simulink model "sampleModel1535"  (R2023a)
settings: Solver=VariableStepAuto  StartTime=0.0  StopTime=10.0  RelTol=1e-3
libraries: simulink x3, hdlsllib x2
settings Model: Creator=user1  LastModifiedBy=user1

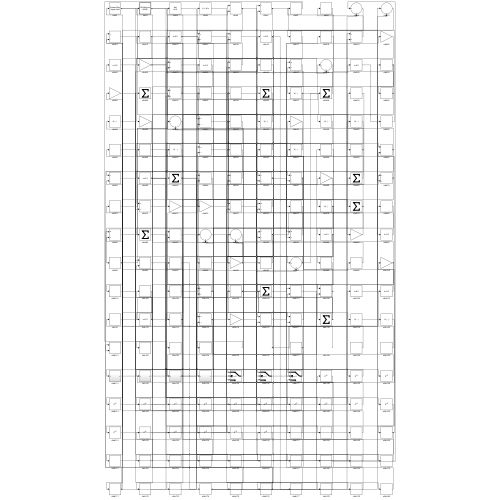
[thumbnail: Simulink's stored preview of the top-level diagram]
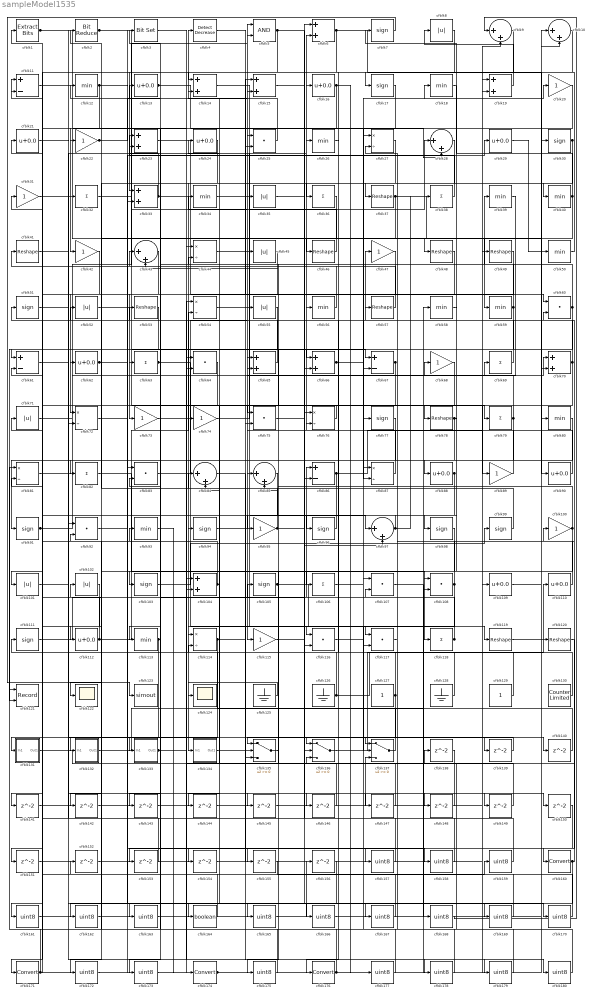
== system sampleModel1535 ==
  cfblk1 : simulink/Logic and Bit Operations/Extract Bits  bitsToExtract=Upper half  numBits=8  bitIdxRange=[0 7]  outScalingMode=Preserve fixed-point scaling
      settings: LibrarySourceBlock=|
      | hdlsllib/Logic and Bit
      | Operations/Extract Bits
  cfblk{9..10,28,43,84..85,97} (7 alike) : Sum  Inputs=|++
  cfblk{20,22,31,42,47,68,73..74,89,95,100,115} (12 alike) : Gain
  cfblk{8,35,45,52,55,71,101..102} (8 alike) : Abs  SaturateOnIntegerOverflow=off
  cfblk{7,17,30,51,77,91,94,96,98..99,103,105,111} (13 alike) : Signum
  cfblk{6,14..15,19,23,33,65..66,70,104} (10 alike) : Sum
  cfblk{32,36,38,63,69,79,82,106,118} (9 alike) : Sum  Inputs=+
  cfblk{25,60,64,75,83,92,107..108,116..117} (10 alike) : DotProduct  OutDataTypeStr=Inherit: Inherit via internal rule
  cfblk{13,16,21,24,29,62,88,90,109..110,112} (11 alike) : Bias  Bias=0.0  SaturateOnIntegerOverflow=off
  cfblk{11,61,67,86} (4 alike) : Sum  Inputs=+-
  cfblk{12,18,26,34,39..40,50,56,58..59,80,93,113} (13 alike) : MinMax
  cfblk{27,44,54,72,76,81,87,114} (8 alike) : Product  Inputs=*/  RndMeth=Zero  SaturateOnIntegerOverflow=on
  cfblk{37,41,46,48..49,53,57,78,119..120} (10 alike) : Reshape
  cfblk121 : Record  FileSettingsInternal="{\"entries\":[{\"content\":{\"excelSettings\":{\"content\":{},\"type\":\"Streamout.ExcelSettings\"}},\"type\":\"Streamout.FileSettingStorage\",\"uuid\":\"\"}],\"packageUris\":[\"http:\\/\\/schema.mathworks.com\\/mf0\\/streamout_blocks\\/R2020a\"],\"version\":\"1.0\"}"  Layout=[1 1]  SignalsInternal="{\"entries\":[{\"content\":{\"signals\":[{\"content\":{\"blockPath\":[],\"dimensions\":[1],\"domain\":\"\",\"lineColor\":\"#a2142f\",\"plots\":[1],\"port\":1,\"signalID\":1564,\"signalName\":\"XY Graph:1\"},\"type\":\"RecordBlkView.Signal\",\"uuid\":\"\"},{\"content\":{\"blockPath\":[],\"dimensions\":[1],\"domain\":\"\",\"lineColor\":\"#139fff\",\"plots\":[1],\"port\":2,\"signalID\":1567,\"signalName\":\"XY Graph:2\"},\"type\":\"RecordBlkView.Signal\",\"uuid\":\"\"}]},\"type\":\"RecordBlkView.InputSignals\",\"uuid\":\"\"}],\"packageUris\":[\"http:\\/\\/schema.mathworks.com\\/mf0\\/streamout_blocks\\/R2020a\"],\"version\":\"1.0\"}"  VisualizationBindings="{\"xyplotplugin\":{\"info\":[{\"series\":[{\"bindingParametersList\":[{\"parameter\":\"X-Axis\",\"signalID\":1564,\"signalName\":\"XY Graph:1\"},{\"parameter\":\"Y-Axis\",\"signalID\":1567,\"signalName\":\"XY Graph:2\"}],\"seriesID\":27336}],\"subplotID\":1}]}}"  CompatibilityTag=XY  st=-1
  cfblk122 : Scope
  cfblk123 : ToWorkspace  VariableName=simout  SaveFormat=Timeseries  SampleTime=-1
  cfblk124 : Scope
  cfblk125 : Ground
  cfblk126 : Ground
  cfblk127 : Constant  SampleTime=-1
  cfblk128 : Ground
  cfblk129 : Constant  SampleTime=-1
  cfblk130 : hdlsllib/Sources/Counter Limited  uplimit=7  tsamp=-1
  cfblk131 : Subsystem
      settings: LibrarySourceBlock=|
      | hdlsllib/Ports &
      | Subsystems/Subsystem
  cfblk132 : Subsystem
      settings: LibrarySourceBlock=|
      | hdlsllib/Ports &
      | Subsystems/Subsystem
  cfblk133 : Subsystem
      settings: LibrarySourceBlock=|
      | hdlsllib/Ports &
      | Subsystems/Subsystem
  cfblk134 : Subsystem
      settings: LibrarySourceBlock=|
      | hdlsllib/Ports &
      | Subsystems/Subsystem
  cfblk135 : Switch  SaturateOnIntegerOverflow=off  InputSameDT=off
  cfblk136 : Switch  SaturateOnIntegerOverflow=off  InputSameDT=off
  cfblk137 : Switch  SaturateOnIntegerOverflow=off  InputSameDT=off
  cfblk{138..156} (19 alike) : Delay  SampleTime=1
  cfblk{157..159,161..163,165..170,172..173,175,177..180} (19 alike) : DataTypeConversion  OutDataTypeStr=uint8  SaturateOnIntegerOverflow=off  RndMeth=Floor
  cfblk{160,171,174,176} (4 alike) : DataTypeConversion  SaturateOnIntegerOverflow=off  RndMeth=Floor
  cfblk164 : DataTypeConversion  OutDataTypeStr=boolean  SaturateOnIntegerOverflow=off  RndMeth=Floor
  cfblk2 : hdlsllib/Logic and Bit Operations/Bit Reduce  mode=AND
  cfblk3 : simulink/Logic and Bit Operations/Bit Set  iBit=0
      settings: LibrarySourceBlock=|
      | hdlsllib/Logic and Bit
      | Operations/Bit Set
  cfblk4 : simulink/Logic and Bit Operations/Detect Decrease  vinit=0.0  OutDataTypeStr=boolean
      settings: LibrarySourceBlock=|
      | hdlsllib/Logic and Bit
      | Operations/Detect
      | Decrease
  cfblk5 : Logic  AllPortsSameDT=off  OutDataTypeStr=boolean
  wires:
  cfblk43/1 -> cfblk73/1
  cfblk130/1 -> cfblk111/1
  cfblk118/1 -> cfblk86/1, cfblk13/1
  cfblk63/1 -> cfblk117/1, cfblk155/1
  cfblk108/1 -> cfblk134/1(In1), cfblk51/1
  cfblk69/1 -> cfblk47/1
  cfblk24/1 -> cfblk114/1
  cfblk131/1(Out1) -> cfblk100/1
  cfblk14/1 -> cfblk116/1
  cfblk7/1 -> cfblk123/1
  cfblk73/1 -> cfblk79/1
  cfblk32/1 -> cfblk48/1
  cfblk28/1 -> cfblk37/1
  cfblk88/1 -> cfblk115/1, cfblk135/2
  cfblk67/1 -> cfblk143/1, cfblk144/1
  cfblk39/1 -> cfblk69/1
  cfblk62/1 -> cfblk148/1, cfblk149/1, cfblk167/1
  cfblk57/1 -> cfblk41/1
  cfblk2/1 -> cfblk89/1, cfblk46/1
  cfblk94/1 -> cfblk5/1
  cfblk120/1 -> cfblk160/1
  cfblk44/1 -> cfblk67/1
  cfblk68/1 -> cfblk96/1
  cfblk106/1 -> cfblk20/1
  cfblk104/1 -> cfblk61/2, cfblk164/1
  cfblk128/1 -> cfblk71/1
  cfblk34/1 -> cfblk97/1
  cfblk23/1 -> cfblk67/2
  cfblk83/1 -> cfblk25/1
  cfblk45/1 -> cfblk63/1
  cfblk96/1 -> cfblk95/1
  cfblk117/1 -> cfblk57/1
  cfblk133/1(Out1) -> cfblk105/1, cfblk178/1
  cfblk71/1 -> cfblk68/1
  cfblk116/1 -> cfblk18/1
  cfblk20/1 -> cfblk42/1
  cfblk29/1 -> cfblk50/1
  cfblk74/1 -> cfblk6/2
  cfblk119/1 -> cfblk80/1
  cfblk27/1 -> cfblk176/1
  cfblk18/1 -> cfblk88/1
  cfblk87/1 -> cfblk65/1
  cfblk91/1 -> cfblk5/2, cfblk11/2
  cfblk1/1 -> cfblk90/1, cfblk135/3
  cfblk103/1 -> cfblk99/1
  cfblk136/1 -> cfblk110/1
  cfblk52/1 -> cfblk77/1
  cfblk81/1 -> cfblk35/1
  cfblk112/1 -> cfblk54/2, cfblk11/1
  cfblk58/1 -> cfblk78/1
  cfblk50/1 -> cfblk17/1
  cfblk17/1 -> cfblk22/1
  cfblk90/1 -> cfblk16/1
  cfblk86/1 -> cfblk19/1, cfblk131/1(In1)
  cfblk95/1 -> cfblk2/1, cfblk119/1
  cfblk33/1 -> cfblk86/2, cfblk23/2
  cfblk19/1 -> cfblk8/1
  cfblk12/1 -> cfblk140/1, cfblk141/1
  cfblk25/1 -> cfblk4/1
  cfblk79/1 -> cfblk45/1, cfblk154/1
  cfblk37/1 -> cfblk59/1, cfblk104/2
  cfblk56/1 -> cfblk43/1
  cfblk36/1 -> cfblk103/1
  cfblk111/1 -> cfblk76/1
  cfblk80/1 -> cfblk82/1
  cfblk16/1 -> cfblk113/1, cfblk177/1
  cfblk137/1 -> cfblk24/1
  cfblk22/1 -> cfblk15/2, cfblk145/1
  cfblk98/1 -> cfblk112/1
  cfblk53/1 -> cfblk121/2
  cfblk93/1 -> cfblk174/1
  cfblk135/1 -> cfblk85/1
  cfblk48/1 -> cfblk122/1
  cfblk15/1 -> cfblk97/2
  cfblk105/1 -> cfblk117/2, cfblk137/2
  cfblk132/1(Out1) -> cfblk58/1
  cfblk78/1 -> cfblk91/1, cfblk108/1
  cfblk76/1 -> cfblk74/1
  cfblk97/1 -> cfblk94/1, cfblk38/1
  cfblk129/1 -> cfblk56/1
  cfblk6/1 -> cfblk33/1, cfblk70/2
  cfblk26/1 -> cfblk136/1
  cfblk113/1 -> cfblk53/1, cfblk172/1
  cfblk4/1 -> cfblk60/1
  cfblk49/1 -> cfblk101/1
  cfblk115/1 -> cfblk136/2
  cfblk82/1 -> cfblk118/1
  cfblk89/1 -> cfblk76/2
  cfblk66/1 -> cfblk87/1, cfblk106/1
  cfblk126/1 -> cfblk65/2, cfblk10/2
  cfblk42/1 -> cfblk72/1
  cfblk38/1 -> cfblk23/1
  cfblk109/1 -> cfblk30/1
  cfblk100/1 -> cfblk43/2, cfblk153/1, cfblk175/1
  cfblk110/1 -> cfblk52/1
  cfblk127/1 -> cfblk137/1, cfblk83/2
  cfblk72/1 -> cfblk29/1
  cfblk9/1 -> cfblk66/1
  cfblk54/1 -> cfblk28/1
  cfblk5/1 -> cfblk61/1, cfblk147/1
  cfblk125/1 -> cfblk124/1
  cfblk10/1 -> cfblk36/1
  cfblk13/1 -> cfblk28/2, cfblk87/2
  cfblk11/1 -> cfblk44/1
  cfblk99/1 -> cfblk84/1
  cfblk64/1 -> cfblk171/1
  cfblk65/1 -> cfblk44/2
  cfblk30/1 -> cfblk62/1, cfblk40/1
  cfblk77/1 -> cfblk84/2
  cfblk8/1 -> cfblk14/1
  cfblk47/1 -> cfblk66/2
  cfblk85/1 -> cfblk133/1(In1)
  cfblk60/1 -> cfblk75/1, cfblk39/1
  cfblk40/1 -> cfblk132/1(In1), cfblk7/1
  cfblk55/1 -> cfblk72/2
  cfblk51/1 -> cfblk32/1
  cfblk101/1 -> cfblk26/1
  cfblk59/1 -> cfblk12/1, cfblk142/1
  cfblk46/1 -> cfblk34/1
  cfblk114/1 -> cfblk70/1, cfblk151/1
  cfblk70/1 -> cfblk98/1, cfblk55/1
  cfblk138/1 -> cfblk136/3
  cfblk41/1 -> cfblk139/1
  cfblk139/1 -> cfblk135/1
  cfblk140/1 -> cfblk114/2
  cfblk141/1 -> cfblk33/2
  cfblk142/1 -> cfblk137/3
  cfblk143/1 -> cfblk54/1
  cfblk144/1 -> cfblk9/2
  cfblk145/1 -> cfblk116/2
  cfblk61/1 -> cfblk146/1
  cfblk146/1 -> cfblk15/1
  cfblk147/1 -> cfblk104/1
  cfblk148/1 -> cfblk85/2
  cfblk149/1 -> cfblk14/2
  cfblk134/1(Out1) -> cfblk150/1
  cfblk151/1 -> cfblk19/2
  cfblk152/1 -> cfblk75/2
  cfblk153/1 -> cfblk1/1
  cfblk154/1 -> cfblk25/2
  cfblk92/1 -> cfblk157/1
  cfblk157/1 -> cfblk6/1
  cfblk75/1 -> cfblk158/1
  cfblk158/1 -> cfblk92/1
  cfblk155/1 -> cfblk159/1
  cfblk159/1 -> cfblk92/2
  cfblk160/1 -> cfblk60/2, cfblk163/1
  cfblk102/1 -> cfblk161/1
  cfblk161/1 -> cfblk120/1
  cfblk156/1 -> cfblk162/1
  cfblk162/1 -> cfblk102/1
  cfblk163/1 -> cfblk156/1
  cfblk164/1 -> cfblk3/1
  cfblk3/1 -> cfblk165/1
  cfblk165/1 -> cfblk109/1
  cfblk21/1 -> cfblk166/1
  cfblk167/1 -> cfblk21/1
  cfblk107/1 -> cfblk168/1
  cfblk168/1 -> cfblk9/1
  cfblk166/1 -> cfblk169/1
  cfblk169/1 -> cfblk107/1
  cfblk35/1 -> cfblk170/1
  cfblk170/1 -> cfblk107/2
  cfblk171/1 -> cfblk81/2, cfblk81/1, cfblk83/1
  cfblk172/1 -> cfblk64/1
  cfblk150/1 -> cfblk173/1
  cfblk173/1 -> cfblk64/2
  cfblk174/1 -> cfblk108/2, cfblk49/1, cfblk10/1
  cfblk175/1 -> cfblk93/1
  cfblk176/1 -> cfblk152/1, cfblk121/1
  cfblk177/1 -> cfblk27/1
  cfblk178/1 -> cfblk27/2
  cfblk31/1 -> cfblk179/1
  cfblk179/1 -> cfblk138/1
  cfblk84/1 -> cfblk180/1
  cfblk180/1 -> cfblk31/1

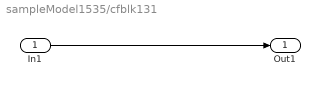
== system sampleModel1535/cfblk131 ==
  In1 : Inport
  Out1 : Outport
  wires:
  In1/1 -> Out1/1

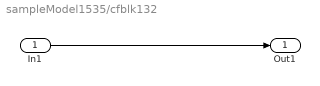
== system sampleModel1535/cfblk132 ==
  In1 : Inport
  Out1 : Outport
  wires:
  In1/1 -> Out1/1

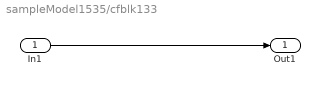
== system sampleModel1535/cfblk133 ==
  In1 : Inport
  Out1 : Outport
  wires:
  In1/1 -> Out1/1

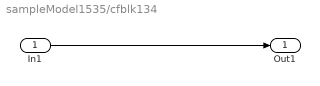
== system sampleModel1535/cfblk134 ==
  In1 : Inport
  Out1 : Outport
  wires:
  In1/1 -> Out1/1
